simulink model "L04_ChristmasLights"  (R2020b)
settings: Solver=FixedStepDiscrete  StartTime=0.0  StopTime=60.0  FixedStep=0.01  RelTol=1e-3
undefined symbols (not defined in the file): sigbuilder_block
settings Model: Creator=ncleju  LastModifiedBy=ncleju

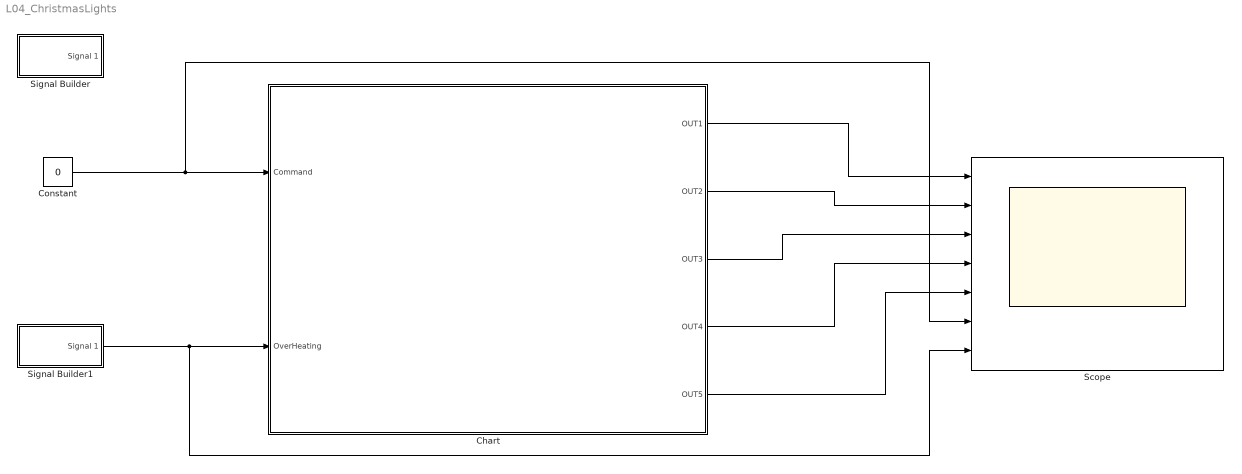
== system L04_ChristmasLights ==
  Chart : Stateflow chart  TreatAsAtomicUnit=on
  Constant : Constant  Value=0
  Scope : Scope  NumInputPorts=7
  Signal Builder : Subsystem  Tag=STV Subsys  LoadFcn=sigbuilder_block('load');  StartFcn=sigbuilder_block('start');  StopFcn=sigbuilder_block('stop');  ClipboardFcn=sigbuilder_block('clipboard');  mask(Sigbuilder block){tuvar=[0:10]}
      mask help: Simulink:masks:SigbuilderBlock_MD
      mask init:
      | if ~strcmp(get_param(bdroot(gcbh),'SimulationStatus'),'stopped') tuvar = sigbuilder_block('maskInit'); end
      settings: CopyFcn=sigbuilder_block('copy');  DeleteFcn=sigbuilder_block('delete');  ModelCloseFcn=sigbuilder_block('modelClose');  PreSaveFcn=sigbuilder_block('preSave');  PauseFcn=sigbuilder_block('pause');  ContinueFcn=sigbuilder_block('continue');  NameChangeFcn=sigbuilder_block('namechange');  OpenFcn=sigbuilder_block('open',[6 30 1428 681.75 ]);  CloseFcn=sigbuilder_block('close');
      mask Display: plot(0, 0, 100, 100,[2, 2, 32, 32, 2], [68, 8, 8, 68, 68],[32, 2], [38, 38], [32, 19, 2],[53, 60, 44], [32, 17, 17, 2],[16, 16, 31, 31]);txt = getActiveGroup(gcbh);text(2, 100, txt,'verticalAlignment', 'top');
  Signal Builder1 : Subsystem  Tag=STV Subsys  LoadFcn=sigbuilder_block('load');  StartFcn=sigbuilder_block('start');  StopFcn=sigbuilder_block('stop');  ClipboardFcn=sigbuilder_block('clipboard');  mask(Sigbuilder block){tuvar=[0:10]}
      mask help: Simulink:masks:SigbuilderBlock_MD
      mask init:
      | if ~strcmp(get_param(bdroot(gcbh),'SimulationStatus'),'stopped') tuvar = sigbuilder_block('maskInit'); end
      settings: CopyFcn=sigbuilder_block('copy');  DeleteFcn=sigbuilder_block('delete');  ModelCloseFcn=sigbuilder_block('modelClose');  PreSaveFcn=sigbuilder_block('preSave');  PauseFcn=sigbuilder_block('pause');  ContinueFcn=sigbuilder_block('continue');  NameChangeFcn=sigbuilder_block('namechange');  OpenFcn=sigbuilder_block('open',[6 30 1428 681.75 ]);  CloseFcn=sigbuilder_block('close');
      mask Display: plot(0, 0, 100, 100,[2, 2, 32, 32, 2], [68, 8, 8, 68, 68],[32, 2], [38, 38], [32, 19, 2],[53, 60, 44], [32, 17, 17, 2],[16, 16, 31, 31]);txt = getActiveGroup(gcbh);text(2, 100, txt,'verticalAlignment', 'top');
  wires:
  Signal Builder1/1(Signal 1) -> Scope/7, Chart/2(OverHeating)
  Chart/1(OUT1) -> Scope/1
  Chart/2(OUT2) -> Scope/2
  Chart/3(OUT3) -> Scope/3
  Chart/4(OUT4) -> Scope/4
  Chart/5(OUT5) -> Scope/5
  Constant/1 -> Scope/6, Chart/1(Command)

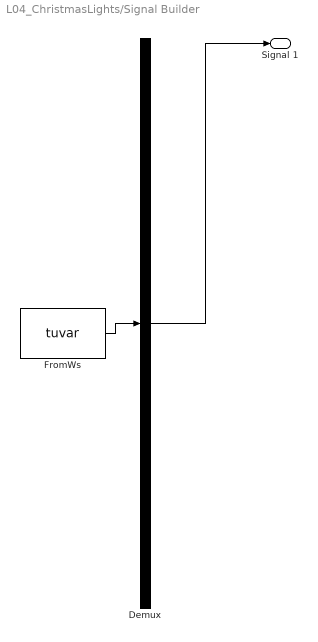
== system L04_ChristmasLights/Signal Builder ==
  Demux : Demux  Tag=STV Demux  Outputs=1
      settings: DisplayOption=none
  FromWs : FromWorkspace  Tag=STV FromWs  VariableName=tuvar
      SigBuilderData=|
      | common.afterFinalStr = 'Extrapolate'
      | common.sampleTime = 0
      | dataSet.timeRange = [0 60]
      | dataSet.name = 'Group 1'
      | sbobj.Groups.Name = 'Group 1'
      | sbobj.Groups.Signals.Name = 'Signal 1'
      | sbobj.Groups.Signals.XData = [0 15.15 15.15 39.1 39.1 60]
      | sbobj.Groups.Signals.YData = [0 0 1 1 0 0]
      | sbobj.Groups.TimeRange = [0 60]
  Signal 1 : Outport  Tag=STV Outport
  wires:
  Demux/1 -> Signal 1/1
  FromWs/1 -> Demux/1

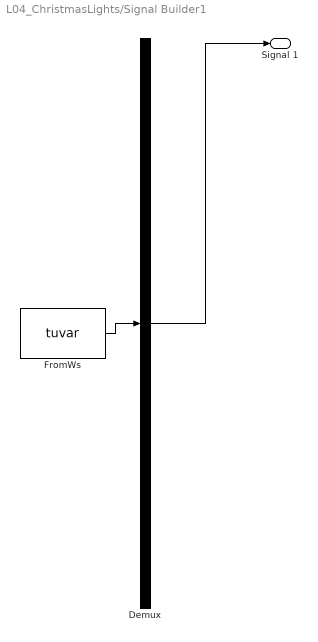
== system L04_ChristmasLights/Signal Builder1 ==
  Demux : Demux  Tag=STV Demux  Outputs=1
      settings: DisplayOption=none
  FromWs : FromWorkspace  Tag=STV FromWs  VariableName=tuvar
      SigBuilderData=|
      | common.afterFinalStr = 'Extrapolate'
      | common.sampleTime = 0
      | dataSet.timeRange = [0 60]
      | dataSet.name = 'Group 1'
      | sbobj.Groups.Name = 'Group 1'
      | sbobj.Groups.Signals.Name = 'Signal 1'
      | sbobj.Groups.Signals.XData = [0 15.35 15.35 36.3 36.3 60]
      | sbobj.Groups.Signals.YData = [0 0 1 1 0 0]
      | sbobj.Groups.TimeRange = [0 60]
  Signal 1 : Outport  Tag=STV Outport
  wires:
  FromWs/1 -> Demux/1
  Demux/1 -> Signal 1/1

== stateflow chart L04_ChristmasLights/Chart ==
  state WORKING
    (history)
    state MODE1
      state FLASH_ON
        en:
        OUT1 = 100;
        OUT2 = 100;
        OUT3 = 100;
        OUT4 = 100;
        OUT5 = 100;
      state FLASH_OFF
        en:
        OUT1 = 0;
        OUT2 = 0;
        OUT3 = 0;
        OUT4 = 0;
        OUT5 = 0;
      (default) -> FLASH_ON
      FLASH_ON -> FLASH_OFF : [after(200, msec)]
      FLASH_OFF -> FLASH_ON : [after(200, msec)]
    state MODE3
      state TRAIN1
        en:
        OUT1 = 100;
        OUT2 = 0;
        OUT3 = 0;
        OUT4 = 0;
        OUT5 = 0;
      state TRAIN2
        en:
        OUT1 = 0;
        OUT2 = 100;
        OUT3 = 0;
        OUT4 = 0;
        OUT5 = 0;
      state TRAIN3
        en:
        OUT1 = 0;
        OUT2 = 0;
        OUT3 = 100;
        OUT4 = 0;
        OUT5 = 0;
      state TRAIN4
        en:
        OUT1 = 0;
        OUT2 = 0;
        OUT3 = 0;
        OUT4 = 100;
        OUT5 = 0;
      state TRAIN5
        en:
        OUT1 = 0;
        OUT2 = 0;
        OUT3 = 0;
        OUT4 = 0;
        OUT5 = 100;
      (default) -> TRAIN1
      TRAIN1 -> TRAIN2 : [after(250,msec)]
      TRAIN3 -> TRAIN4 : [after(250,msec)]
      TRAIN4 -> TRAIN5 : [after(250,msec)]
      TRAIN2 -> TRAIN3 : [after(250,msec)]
      TRAIN5 -> TRAIN1 : [after(250,msec)]
    state MODE2
      state INCR
      state DECR
      (default) -> INCR : {OUT1 = 0;
          | OUT2 = 0;
          | OUT3 = 0;
          | OUT4 = 0;
          | OUT5 = 0;}
      INCR -> INCR [order 1] : [after(30, msec)]
          | {OUT1 = OUT1+1;
          | OUT2 = OUT2+1;
          | OUT3 = OUT3+1;
          | OUT4 = OUT4+1;
          | OUT5 = OUT5+1;}
      INCR -> DECR [order 2] : [OUT1 == 100]
          | {OUT1 = 100;
          | OUT2 = 100;
          | OUT3 = 100;
          | OUT4 = 100;
          | OUT5 = 100;}
      DECR -> INCR [order 2] : [OUT1 == 0]
          | {OUT1 = 0;
          | OUT2 = 0;
          | OUT3 = 0;
          | OUT4 = 0;
          | OUT5 = 0;}
      DECR -> DECR [order 1] : [after(30, msec)]
          | {OUT1 = OUT1-1;
          | OUT2 = OUT2-1;
          | OUT3 = OUT3-1;
          | OUT4 = OUT4-1;
          | OUT5 = OUT5-1;}
    (default) -> MODE1
    MODE3 -> MODE1 [order 1] : [after(10,sec) && Command==0]
    MODE3 -> MODE1 [order 2] : [Command==1]
    MODE1 -> MODE3 [order 3] : [Command==3]
    MODE1 -> MODE2 [order 1] : [after(10,sec) && Command==0]
    MODE2 -> MODE1 [order 2] : [Command==1]
    MODE1 -> MODE2 [order 2] : [Command==2]
    MODE3 -> MODE2 [order 3] : [Command==2]
    MODE2 -> MODE3 [order 3] : [Command==3]
    MODE2 -> MODE3 [order 1] : [after(10,sec) && Command==0]
  state PAUSE
    en:
    OUT1 = 0;
    OUT2 = 0;
    OUT3 = 0;
    OUT4 = 0;
    OUT5 = 0;
  (default) -> WORKING
  WORKING -> PAUSE : [OverHeating == true]
  PAUSE -> WORKING : [after(15, sec) && OverHeating == false]
  data: Command input; OverHeating input; OUT1 output; OUT2 output; OUT3 output; OUT4 output; OUT5 output
